simulink model "withoutDOB"  (R2017a)
settings: Solver=VariableStepAuto  StartTime=0.0  StopTime=10.0  RelTol=1e-3
libraries: cstblocks x2
settings Model: Creator=15062  LastModifiedBy=15062

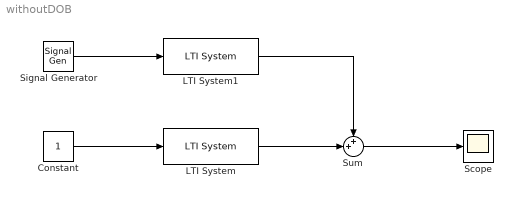
== system withoutDOB ==
  Constant : Constant
  LTI System : cstblocks/LTI System  sys=Gd1  IC=[]
  LTI System1 : cstblocks/LTI System  sys=Gd2  IC=[]
  Scope : Scope
  Signal Generator : SignalGenerator  Units=rad/sec
  Sum : Sum  Inputs=++|
  wires:
  Signal Generator/1 -> LTI System1/1
  LTI System/1 -> Sum/2
  LTI System1/1 -> Sum/1
  Sum/1 -> Scope/1
  Constant/1 -> LTI System/1
